simulink model "invdyncontrolOBS1"  (Simulink 7.4)
settings: Solver=ode23s  StartTime=0.0  StopTime=4  MinStep=1e-3  RelTol=1e-3
undefined symbols (not defined in the file or in its folder): inertcalc, ncalc, observer, selectde, selectdx1e, selectdx2e
libraries: roblocks x2
settings Model: Creator=acolome  LastModifiedBy=acolome

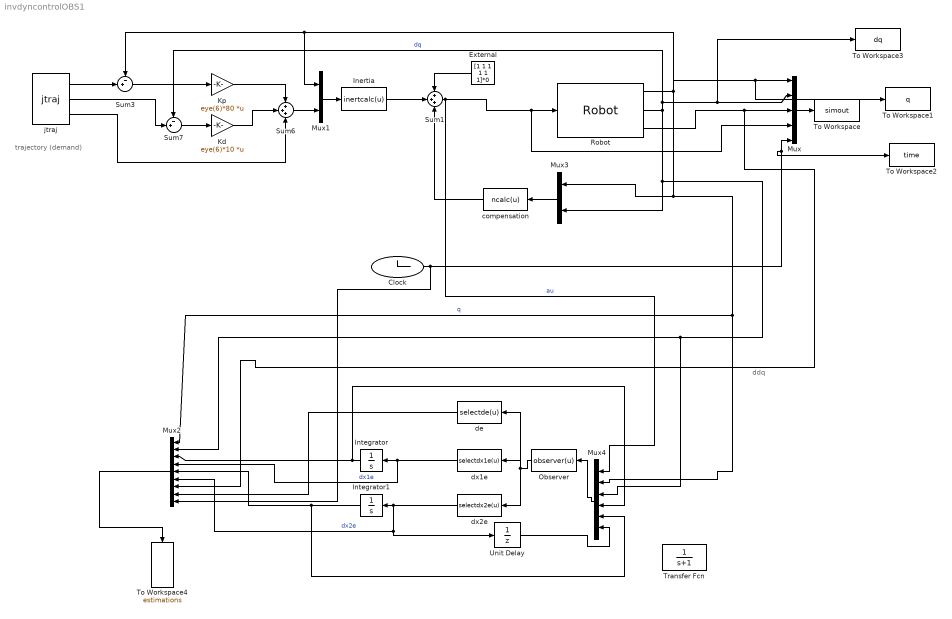
== system invdyncontrolOBS1 ==
  note: trajectory
      | (demand)
  note: ddq
  Clock : Clock
      settings: Decimation=100
  External : Constant  Value=[1 1 1 1 1 1]*0  OutDataType=fixdt(1, 16)  OutScaling=2^0
  Inertia : MATLABFcn  MATLABFcn=inertcalc(u)
  Integrator : Integrator  InitialCondition=[0 0 0 0 0 0]
  Integrator1 : Integrator  InitialCondition=[0 0 0 0 0 0]
  Kd : Gain  Gain=eye(6)*10  Multiplication=Matrix(K*u)  SaturateOnIntegerOverflow=on  OutDataTypeStr=Inherit: Same as input  ParamDataTypeStr=Inherit: Same as input
  Kp : Gain  Gain=eye(6)*80  Multiplication=Matrix(K*u)  SaturateOnIntegerOverflow=on  OutDataTypeStr=Inherit: Same as input  ParamDataTypeStr=Inherit: Same as input
  Mux : Mux  Inputs=5
  Mux1 : Mux  Inputs=2
  Mux2 : Mux  Inputs=9
  Mux3 : Mux  Inputs=2
  Mux4 : Mux  Inputs=6
  Observer : MATLABFcn  MATLABFcn=observer(u)
  Robot : roblocks/Robot  SystemSampleTime=-1  robot=p560  q0=[0 0 0 0 0 0]
  Sum1 : Sum  Inputs=+++  OutDataType=fixdt(1, 16)  OutScaling=2^0
  Sum3 : Sum  Inputs=-+|  SaturateOnIntegerOverflow=on  InputSameDT=on  OutDataTypeStr=Inherit: Same as first input
  Sum6 : Sum  Inputs=+++  OutDataType=fixdt(1, 16)  OutScaling=2^0
  Sum7 : Sum  Inputs=-+|  SaturateOnIntegerOverflow=on  InputSameDT=on  OutDataTypeStr=Inherit: Same as first input
  To Workspace : ToWorkspace  VariableName=simout  SampleTime=-1  SaveFormat=Array
  To Workspace1 : ToWorkspace  VariableName=q  SampleTime=-1  SaveFormat=Array
  To Workspace2 : ToWorkspace  VariableName=time  SampleTime=-1  SaveFormat=Array
  To Workspace3 : ToWorkspace  VariableName=dq  SampleTime=-1  SaveFormat=Array
  To Workspace4 : ToWorkspace  VariableName=estimations  SampleTime=-1  SaveFormat=Array
  Transfer Fcn : TransferFcn  Denominator=[1 1]
  Unit Delay : UnitDelay  X0=[0 0 0 0 0 0]  SampleTime=0
  compensation : MATLABFcn  MATLABFcn=ncalc(u)
  de : MATLABFcn  MATLABFcn=selectde(u)
  dx1e : MATLABFcn  MATLABFcn=selectdx1e(u)
  dx2e : MATLABFcn  MATLABFcn=selectdx2e(u)
  jtraj : roblocks/jtraj  SystemSampleTime=-1  q0=[pi/4 pi/2 -pi/2 0 0 0]*0  qf=[1 1 1 1 1 1]  tmax=4
      link override MATLAB Fcn: MATLABFcn=squeeze(interp1(t,q,u))
      link override MATLAB Fcn1: MATLABFcn=squeeze(interp1(t,qd,u))
      link override MATLAB Fcn2: MATLABFcn=squeeze(interp1(t,qdd,u))
  wires:
  Mux/1 -> To Workspace/1
  jtraj/2 -> Sum7/2
  Sum7/1 -> Kd/1
  Sum3/1 -> Kp/1
  jtraj/3 -> Sum6/3
  Kd/1 -> Sum6/2
  Kp/1 -> Sum6/1
  jtraj/1 -> Sum3/2
  Robot/1 -> Sum3/1, Mux1/1, Mux/1, To Workspace1/1, Mux2/1, Mux4/2, Mux3/1  "q"
  Robot/2 -> Sum7/1, Mux/2, To Workspace3/1, Mux3/2, Mux2/2, Mux4/3  "dq"
  Mux1/1 -> Inertia/1
  Sum6/1 -> Mux1/2
  Sum1/1 -> Robot/1, Mux/4, Mux4/1  "au"
  Mux3/1 -> compensation/1
  Robot/3 -> Mux/3, Mux2/7
  Clock/1 -> Mux/5, To Workspace2/1, Mux2/9
  Mux2/1 -> To Workspace4/1
  Mux4/1 -> Observer/1
  Observer/1 -> de/1, dx2e/1, dx1e/1
  Integrator1/1 -> Mux2/5, Mux4/5
  Integrator/1 -> Mux2/3, Mux4/4
  compensation/1 -> Sum1/3
  Inertia/1 -> Sum1/2
  External/1 -> Sum1/1
  Unit Delay/1 -> Mux4/6
  de/1 -> Mux2/8
  dx1e/1 -> Integrator/1, Mux2/4  "dx1e"
  dx2e/1 -> Integrator1/1, Mux2/6, Unit Delay/1  "dx2e"
